simulink model "theta_axis_model"  (R2024b)
settings: Solver=ode4  StartTime=0.0  StopTime=simulation_time  FixedStep=Ts  RelTol=1e-3
undefined symbols (not defined in the file): b_theta, ff_enable, J_theta, Kd_theta, Ki_theta, Kp_theta, move_time, T_theta_max, theta_final, theta_initial, Ts
libraries: slpidlib x1
settings Model: Creator=dell  LastModifiedBy=dell

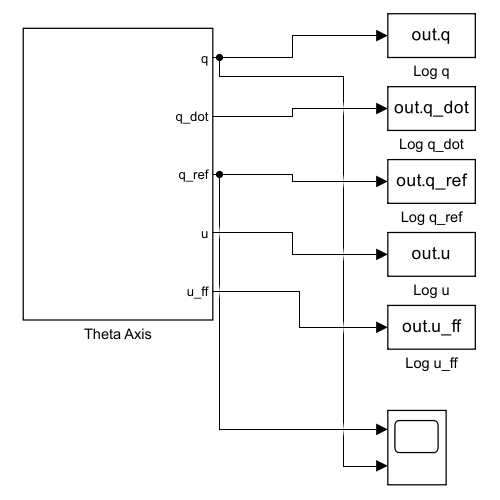
[thumbnail: Simulink's stored preview of the top-level diagram]
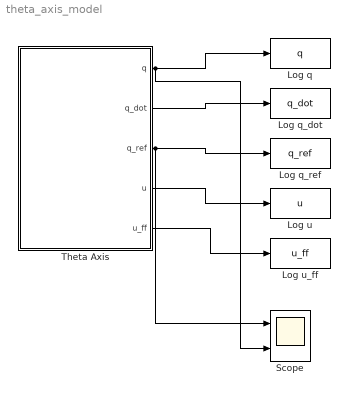
== system theta_axis_model ==
  Log q : ToWorkspace  VariableName=q  SaveFormat=Timeseries  SampleTime=-1
  Log q_dot : ToWorkspace  VariableName=q_dot  SaveFormat=Timeseries  SampleTime=-1
  Log q_ref : ToWorkspace  VariableName=q_ref  SaveFormat=Timeseries  SampleTime=-1
  Log u : ToWorkspace  VariableName=u  SaveFormat=Timeseries  SampleTime=-1
  Log u_ff : ToWorkspace  VariableName=u_ff  SaveFormat=Timeseries  SampleTime=-1
  Scope : Scope  NumInputPorts=2
  Theta Axis : Subsystem
  wires:
  Theta Axis/1(q) -> Log q/1, Scope/2
  Theta Axis/2(q_dot) -> Log q_dot/1
  Theta Axis/3(q_ref) -> Log q_ref/1, Scope/1
  Theta Axis/4(u) -> Log u/1
  Theta Axis/5(u_ff) -> Log u_ff/1

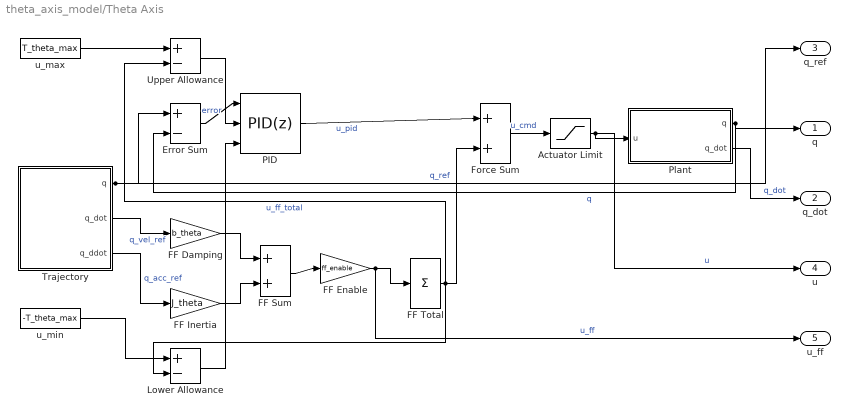
== system theta_axis_model/Theta Axis ==
  Actuator Limit : Saturate  UpperLimit=T_theta_max  LowerLimit=-T_theta_max
  Error Sum : Sum  Inputs=+-
  FF Damping : Gain  Gain=b_theta
  FF Enable : Gain  Gain=ff_enable
  FF Inertia : Gain  Gain=J_theta
  FF Sum : Sum
  FF Total : Sum  Inputs=+
  Force Sum : Sum
  Lower Allowance : Sum  Inputs=+-
  PID : slpidlib/PID Controller  Controller=PID  Form=Parallel  TimeDomain=Discrete-time  UseExternalTs=off  SampleTime=Ts  IntegratorMethod=Backward Euler  FilterMethod=Forward Euler  ControllerParametersSource=internal  P=Kp_theta  I=Ki_theta  UseKiTs=off  D=Kd_theta  UseExternalDerivativeSource=off  N=100  UseFilter=off  TunerSelectOption=Transfer Function Based (PID Tuner App)  InitialConditionSource=internal  InitialConditionForIntegrator=0  InitialConditionForFilter=0  DifferentiatorICPrevScaledInput=0  ExternalReset=none  TrackingMode=off  Kt=1  LimitOutput=on  SatLimitsSource=external  UpperSaturationLimit=inf  LowerSaturationLimit=-inf  LinearizeAsGain=off  AntiWindupMode=clamping  Kb=1  LimitIntegrator=off  UpperIntegratorSaturationLimit=inf  LowerIntegratorSaturationLimit=-inf  POutMin=[]  POutMax=[]  IOutMin=[]  IOutMax=[]  DOutMin=[]  DOutMax=[]  NOutMin=[]  NOutMax=[]  SumOutMin=[]  SumOutMax=[]  SaturationOutMin=[]  SaturationOutMax=[]  PParamMin=[]  PParamMax=[]  IParamMin=[]  IParamMax=[]  DParamMin=[]  DParamMax=[]  NParamMin=[]  NParamMax=[]  KbParamMin=[]  KbParamMax=[]  KtParamMin=[]  KtParamMax=[]  KbOutMin=[]  KbOutMax=[]  KtOutMin=[]  KtOutMax=[]  IntegratorOutMin=[]  IntegratorOutMax=[]  FilterOutMin=[]  FilterOutMax=[]  SumI1OutMin=[]  SumI1OutMax=[]  SumI2OutMin=[]  SumI2OutMax=[]  SumI3OutMin=[]  SumI3OutMax=[]  SumI4OutMin=[]  SumI4OutMax=[]  SumDOutMin=[]  SumDOutMax=[]  DifferentiatorOutMin=[]  DifferentiatorOutMax=[]  FilterDiffOutCoefMin=[]  FilterDiffOutCoefMax=[]  ReciprocalOutMin=[]  ReciprocalOutMax=[]  SumDenOutMin=[]  SumDenOutMax=[]  SumNumOutMin=[]  SumNumOutMax=[]  DivideOutMin=[]  DivideOutMax=[]  UdiffTsProdOutMin=[]  UdiffTsProdOutMax=[]  NTsProdOutMin=[]  NTsProdOutMax=[]  UintegralTsProdOutMin=[]  UintegralTsProdOutMax=[]  UngainTsProdOutMin=[]  UngainTsProdOutMax=[]  ClampingZeroOutDataTypeStr=Inherit: Inherit via back propagation  ClampingZeroOutMin=[]  ClampingZeroOutMax=[]  FilterDenConstantOutDataTypeStr=Inherit: Inherit via back propagation  FilterDenConstantOutMin=[]  FilterDenConstantOutMax=[]  PCopyOutDataTypeStr=Inherit: Inherit via back propagation  PCopyOutMin=[]  PCopyOutMax=[]  NCopyOutDataTypeStr=Inherit: Inherit via back propagation  NCopyOutMin=[]  NCopyOutMax=[]  IntegratorContinuousStateAttributes=''  IntegratorStateMustResolveToSignalObject=off  IntegratorRTWStateStorageClass=Auto  FilterContinuousStateAttributes=''  FilterStateMustResolveToSignalObject=off  FilterRTWStateStorageClass=Auto  ParallelPVariant=InternalParameters  IdealPVariant=Disabled  IVariant=InternalParameters  DVariant=InternalParameters  IntegratorVariant=Discrete  SatVariant=External  AWVariant=DiscClampingParallel  PCopyVariant=Disabled  TRVariant=Disabled  FdbkBlocksVariant=Feedback  IdealPFdbkVariant=Passthrough  SatFdbkVariant=Passthrough  DerivativeFilterVariant=Differentiator  NVariant=Passthrough  NCopyVariant=Disabled_SignalSpec  FilterICVariant=InternalICsDifferentiator  IntegratorICVariant=InternalICs  ExternalResetVariant=Disabled  TRSumVariant=Passthrough  SumFdbkVariant=Enabled  SumVariant=Sum_PID  TsampFilterVariant=InternalTs  TsampNgainVariant=Passthrough  TsampIntegralVariant=Disabled_SignalSpec  ExternalSaturationOutDataTypeStr=Inherit: Same as second input  DerivativeSourceVariant=ErrorSignal  PreIntVariant=InternalPreInt
      settings: LibrarySourceBlock=simulink/Discrete/Discrete PID Controller
  Plant : Subsystem
  Trajectory : Subsystem  mask(Quintic Trajectory){q0=theta_initial, qf=theta_final, T=move_time}
      mask prompts: q0 "Start position q0"; qf "Final position qf"; T "Duration T (s)"
      mask help: Rest-to-rest quintic trajectory from q0 to qf over T seconds. Outputs position, velocity and acceleration.
      mask Display: disp('Quintic Trajectory')
  Upper Allowance : Sum  Inputs=+-
  u_max : Constant  Value=T_theta_max
  u_min : Constant  Value=-T_theta_max
  q : Outport
  q_dot : Outport  Port=2
  q_ref : Outport  Port=3
  u : Outport  Port=4
  u_ff : Outport  Port=5
  wires:
  Trajectory/1(q) -> Error Sum/1, q_ref/1  "q_ref"
  Trajectory/2(q_dot) -> FF Damping/1  "q_vel_ref"
  Trajectory/3(q_ddot) -> FF Inertia/1  "q_acc_ref"
  FF Damping/1 -> FF Sum/1
  FF Inertia/1 -> FF Sum/2
  FF Sum/1 -> FF Enable/1
  FF Enable/1 -> FF Total/1, u_ff/1  "u_ff"
  Error Sum/1 -> PID/1  "error"
  PID/1 -> Force Sum/1  "u_pid"
  FF Total/1 -> Force Sum/2, Upper Allowance/2, Lower Allowance/2  "u_ff_total"
  u_max/1 -> Upper Allowance/1
  u_min/1 -> Lower Allowance/1
  Upper Allowance/1 -> PID/2
  Lower Allowance/1 -> PID/3
  Force Sum/1 -> Actuator Limit/1  "u_cmd"
  Actuator Limit/1 -> Plant/1(u), u/1  "u"
  Plant/1(q) -> q/1, Error Sum/2  "q"
  Plant/2(q_dot) -> q_dot/1  "q_dot"

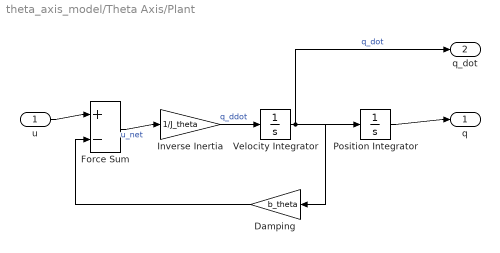
== system theta_axis_model/Theta Axis/Plant ==
  u : Inport
  Damping : Gain  Gain=b_theta
  Force Sum : Sum  Inputs=+-
  Inverse Inertia : Gain  Gain=1/J_theta
  Position Integrator : Integrator  InitialCondition=theta_initial
  Velocity Integrator : Integrator
  q : Outport
  q_dot : Outport  Port=2
  wires:
  u/1 -> Force Sum/1
  Force Sum/1 -> Inverse Inertia/1  "u_net"
  Inverse Inertia/1 -> Velocity Integrator/1  "q_ddot"
  Velocity Integrator/1 -> Position Integrator/1, Damping/1, q_dot/1  "q_dot"
  Damping/1 -> Force Sum/2
  Position Integrator/1 -> q/1

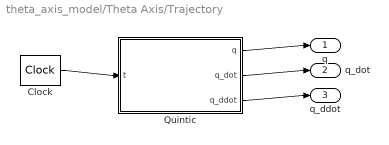
== system theta_axis_model/Theta Axis/Trajectory ==
  Clock : DigitalClock  SampleTime=Ts
  Quintic : MATLAB Function  TreatAsAtomicUnit=on
  q : Outport
  q_dot : Outport  Port=2
  q_ddot : Outport  Port=3
  wires:
  Clock/1 -> Quintic/1(t)
  Quintic/1(q) -> q/1
  Quintic/2(q_dot) -> q_dot/1
  Quintic/3(q_ddot) -> q_ddot/1

== matlab function theta_axis_model/Theta Axis/Trajectory/Quintic ==
  data: t input; q output; q_dot output; q_ddot output; q0 parameter; qf parameter; T parameter
function [q, q_dot, q_ddot] = quintic(t, q0, qf, T)
% Rest-to-rest quintic: zero velocity and acceleration at both ends
tau = min(max(t / T, 0), 1);
d = qf - q0;
q = q0 + d * (10*tau^3 - 15*tau^4 + 6*tau^5);
q_dot = d / T * (30*tau^2 - 60*tau^3 + 30*tau^4);
q_ddot = d / T^2 * (60*tau - 180*tau^2 + 120*tau^3);
